simulink model "without_acceleration"  (R2021a)
settings: Solver=VariableStepAuto  StartTime=0.0  StopTime=10.0  RelTol=1e-3
settings Model: Creator=Osman  LastModifiedBy=Osman

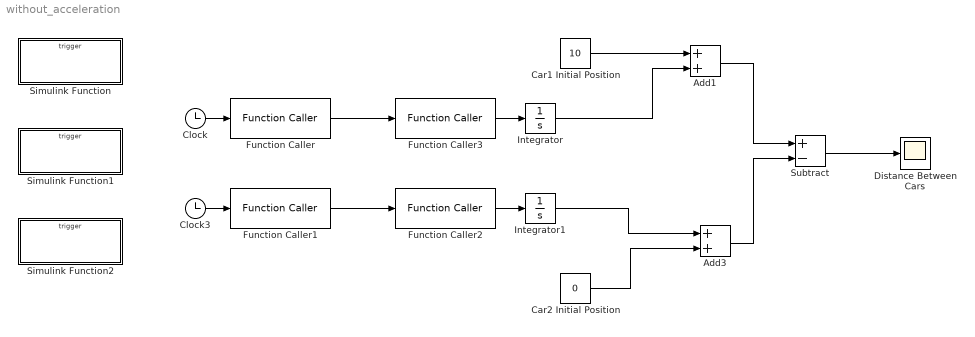
== system without_acceleration ==
  Add1 : Sum
  Add3 : Sum  OutDataTypeStr=double
  Car1 Initial Position : Constant  Value=10
  Car2 Initial Position : Constant  Value=0
  Clock : Clock
  Clock3 : Clock
  Distance Between Cars : Scope
  Function Caller : FunctionCaller  FunctionPrototype=y = vel1(u)  InputArgumentSpecifications=<Enter example>  OutputArgumentSpecifications=<Enter example>
  Function Caller1 : FunctionCaller  FunctionPrototype=y = vel2(u)  InputArgumentSpecifications=<Enter example>  OutputArgumentSpecifications=<Enter example>
  Function Caller2 : FunctionCaller  FunctionPrototype=y = vel_conv(u)  InputArgumentSpecifications=<Enter example>  OutputArgumentSpecifications=<Enter example>
  Function Caller3 : FunctionCaller  FunctionPrototype=y = vel_conv(u)  InputArgumentSpecifications=<Enter example>  OutputArgumentSpecifications=<Enter example>
  Integrator : Integrator
  Integrator1 : Integrator
  Simulink Function : Subsystem  TreatAsAtomicUnit=on
  Simulink Function1 : Subsystem  TreatAsAtomicUnit=on
  Simulink Function2 : Subsystem  TreatAsAtomicUnit=on
  Subtract : Sum  Inputs=+-  OutDataTypeStr=double
  wires:
  Clock/1 -> Function Caller/1
  Function Caller/1 -> Function Caller3/1
  Car1 Initial Position/1 -> Add1/1
  Function Caller1/1 -> Function Caller2/1
  Car2 Initial Position/1 -> Add3/2
  Add1/1 -> Subtract/1
  Add3/1 -> Subtract/2
  Subtract/1 -> Distance Between Cars/1
  Clock3/1 -> Function Caller1/1
  Function Caller3/1 -> Integrator/1
  Function Caller2/1 -> Integrator1/1
  Integrator/1 -> Add1/2
  Integrator1/1 -> Add3/1

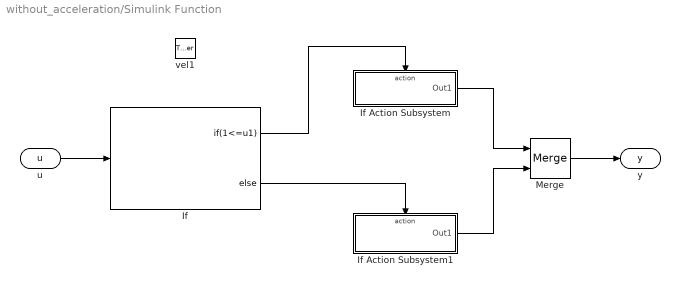
== system without_acceleration/Simulink Function ==
  vel1 : TriggerPort  TriggerType=function-call  IsSimulinkFunction=on  FunctionName=vel1  FunctionVisibility=scoped  VariantControl=(inherit)
  If : If  IfExpression=1<=u1
  If Action Subsystem : Subsystem  TreatAsAtomicUnit=on
  If Action Subsystem1 : Subsystem  TreatAsAtomicUnit=on
  Merge : Merge
  u : ArgIn  DisableCoverage=on  ArgumentName=u
  y : ArgOut  DisableCoverage=on  ArgumentName=y
  wires:
  If/1 -> If Action Subsystem/Action
  If Action Subsystem/1(Out1) -> Merge/1
  If Action Subsystem1/1(Out1) -> Merge/2
  If/2 -> If Action Subsystem1/Action
  u/1 -> If/1
  Merge/1 -> y/1

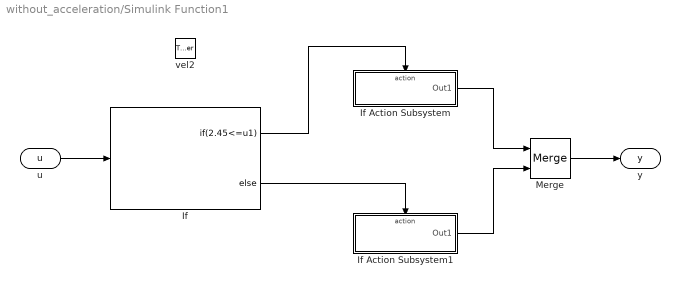
== system without_acceleration/Simulink Function1 ==
  vel2 : TriggerPort  TriggerType=function-call  IsSimulinkFunction=on  FunctionName=vel2  FunctionVisibility=scoped  VariantControl=(inherit)
  If : If  IfExpression=2.45<=u1
  If Action Subsystem : Subsystem  TreatAsAtomicUnit=on
  If Action Subsystem1 : Subsystem  TreatAsAtomicUnit=on
  Merge : Merge
  u : ArgIn  DisableCoverage=on  ArgumentName=u
  y : ArgOut  DisableCoverage=on  ArgumentName=y
  wires:
  If/1 -> If Action Subsystem/Action
  If Action Subsystem/1(Out1) -> Merge/1
  If Action Subsystem1/1(Out1) -> Merge/2
  If/2 -> If Action Subsystem1/Action
  u/1 -> If/1
  Merge/1 -> y/1

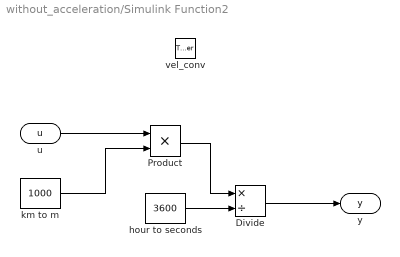
== system without_acceleration/Simulink Function2 ==
  vel_conv : TriggerPort  TriggerType=function-call  IsSimulinkFunction=on  FunctionName=vel_conv  FunctionVisibility=scoped  VariantControl=(inherit)
  Divide : Product  Inputs=*/
  Product : Product
  hour to seconds : Constant  Value=3600
  km to m : Constant  Value=1000
  u : ArgIn  DisableCoverage=on  ArgumentName=u
  y : ArgOut  DisableCoverage=on  ArgumentName=y
  wires:
  u/1 -> Product/1
  km to m/1 -> Product/2
  hour to seconds/1 -> Divide/2
  Product/1 -> Divide/1
  Divide/1 -> y/1

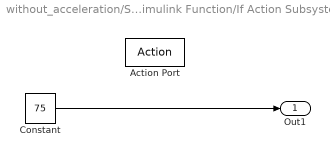
== system without_acceleration/Simulink Function/If Action Subsystem ==
  Action Port : ActionPort  ActionPortLabel=if(1<=u1)
  Constant : Constant  Value=75
  Out1 : Outport
  wires:
  Constant/1 -> Out1/1

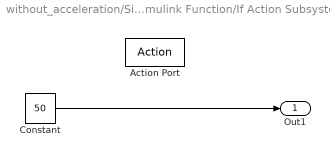
== system without_acceleration/Simulink Function/If Action Subsystem1 ==
  Action Port : ActionPort  ActionPortLabel=else
  Constant : Constant  Value=50
  Out1 : Outport
  wires:
  Constant/1 -> Out1/1

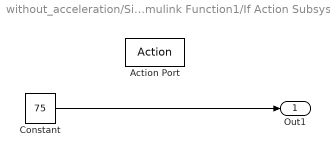
== system without_acceleration/Simulink Function1/If Action Subsystem ==
  Action Port : ActionPort  ActionPortLabel=if(2.45<=u1)
  Constant : Constant  Value=75
  Out1 : Outport
  wires:
  Constant/1 -> Out1/1

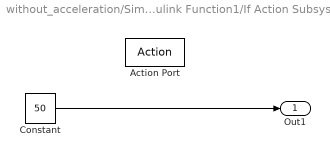
== system without_acceleration/Simulink Function1/If Action Subsystem1 ==
  Action Port : ActionPort  ActionPortLabel=else
  Constant : Constant  Value=50
  Out1 : Outport
  wires:
  Constant/1 -> Out1/1
